simulink model "udpsndrcv"  (R2018b)
settings: Solver=ode4  StartTime=0.0  StopTime=inf  FixedStep=1/500  RelTol=1e-3
libraries: instrumentlib x2, vrlib x1
settings Model: Creator=pprz  LastModifiedBy=pprz
settings DebuggingCC: LibraryContextMissingDiagnostic=none
settings SFSimCC: SimUseLocalCustomCode=off
settings RTWCC: RTWUseLocalCustomCode=off

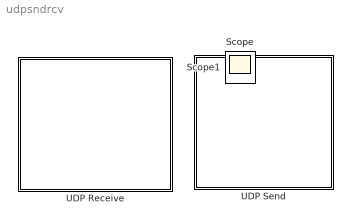
== system udpsndrcv ==
  UDP Receive : Subsystem
  UDP Send : Subsystem
  Scope : Scope
  Scope1 : Scope

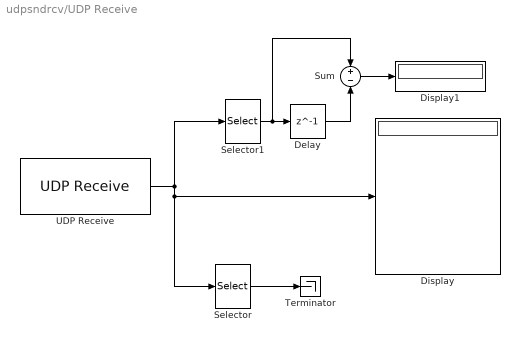
== system udpsndrcv/UDP Receive ==
  Delay : Delay  DelayLength=1
  Display : Display
  Display1 : Display
  Selector : Selector  InputPortWidth=8  IndexOptions=Index vector (dialog)  Indices=[3 4 5]  OutputSizes=1
  Selector1 : Selector  InputPortWidth=8  IndexOptions=Index vector (dialog)  Indices=[2]  OutputSizes=1
  Sum : Sum  Inputs=+-
  Terminator : Terminator
  UDP Receive : instrumentlib/UDP Receive  Host=localhost  Port=9090  LocalPort=5005  EnablePortSharing=off  GetLatestData=off  DataSize="[1  8]"  DataType=ASCII  ASCIIFormatting=%f  Terminator=LF  ByteOrder=BigEndian  EnableBlockingMode=on  Timeout=10  SampleTime=-1  LocalAddress=localhost
      settings: SourceProductName=Instrument Control Toolbox
  wires:
  UDP Receive/1 -> Display/1, Selector/1, Selector1/1
  Selector/1 -> Terminator/1
  Selector1/1 -> Sum/1, Delay/1
  Delay/1 -> Sum/2
  Sum/1 -> Display1/1

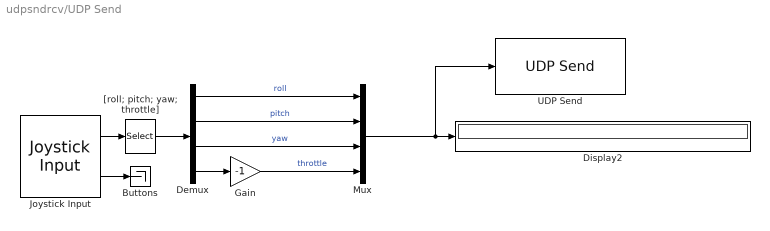
== system udpsndrcv/UDP Send ==
  Buttons : Terminator
  Demux : Demux
  Display2 : Display
  Gain : Gain  Gain=-1
  Joystick Input : vrlib/Joystick Input  joyid=1  adjustports=on  forcefeed=off
      settings: SourceProductBaseCode=VR
  Mux : Mux
  UDP Send : instrumentlib/UDP Send  Host=localhost  Port=9090  LocalPort=-1  EnablePortSharing=off  ByteOrder=BigEndian  OutputDatagramPacketSize=512  EnableBlockingMode=on  LocalAddress=0.0.0.0
      settings: SourceProductName=Instrument Control Toolbox
  "[roll; pitch; yaw; throttle]" : Selector  InputPortWidth=6  IndexOptions=Index vector (dialog)  Indices=[1 2 3 4]  OutputSizes=1
  wires:
  Joystick Input/2 -> Buttons/1
  Demux/1 -> Mux/1  "roll"
  Demux/2 -> Mux/2  "pitch"
  Gain/1 -> Mux/4  "throttle"
  Demux/4 -> Gain/1
  Demux/3 -> Mux/3  "yaw"
  Joystick Input/1 -> "[roll; pitch; yaw; throttle]"/1
  "[roll; pitch; yaw; throttle]"/1 -> Demux/1
  Mux/1 -> UDP Send/1, Display2/1
